simulink model "Comparacion"  (R2018a)
settings: Solver=VariableStepAuto  StartTime=0.0  StopTime=500  FixedStep=0.5  RelTol=1e-3
values from neighbouring files (symbols this model uses):
  A = [S.A zeros(n,p); -S.C eye(p)]    [poles_int.m]
  B = [S.B; zeros(p,m)]    [poles_int.m]
  q0 = eval(solucionParam.qs0)    [discretizacion.m]
  q1 = eval(solucionParam.qs1)    [discretizacion.m]
  q2 = eval(solucionParam.qs2)    [discretizacion.m]
  r1 = eval(solucionParam.rs1)    [discretizacion.m]
  ro = 0.0683    [LaplaceAzeta.m]    (also in discretizacion.m = 0.0683238685925)
  saturMax = 2    [discretizacion.m]
  saturMin = -.5    (= -0.5)    [discretizacion.m]
  so = 0.3356    [LaplaceAzeta.m]    (also in discretizacion.m = 0.335599308431)
  uo = 0.12    [LaplaceAzeta.m]    (also in discretizacion.m)
libraries: simulink x4
settings Model: Creator=posoriol1  LastModifiedBy=posoriol1

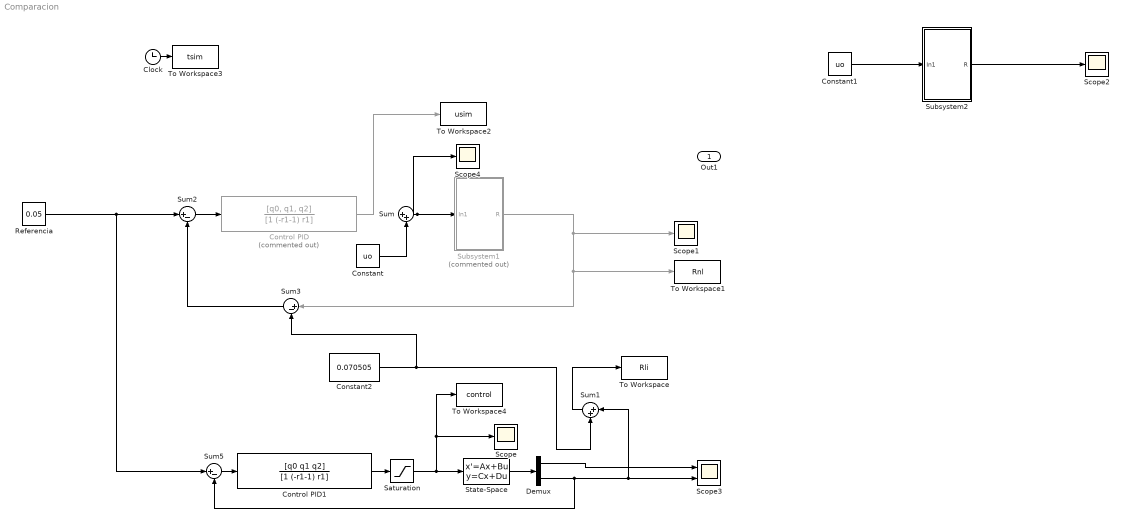
== system Comparacion ==
  Clock : Clock
  Constant : Constant  Value=uo  SampleTime=0.5
  Constant1 : Constant  Value=uo
  Constant2 : Constant  Value=0.070505
  Control PID : DiscreteTransferFcn  Commented=on  Numerator=[q0, q1, q2]  Denominator=[1 (-r1-1) r1]  SampleTime=0.5
  Control PID1 : DiscreteTransferFcn  Numerator=[q0 q1 q2]  Denominator=[1 (-r1-1) r1]  SampleTime=0.5
  Demux : Demux  Outputs=2
  Referencia : Constant  Value=0.05  SampleTime=0.5
  Saturation : Saturate  UpperLimit=saturMax  LowerLimit=saturMin
  Scope{,1..2,4} (4 alike) : Scope
  Scope3 : Scope  NumInputPorts=2
  State-Space : StateSpace  A=A  B=B  C=[1 0; 0 1]  D=[ 0;0]  InitialCondition=0
  Subsystem1 : Subsystem  Commented=on  mask{par=[0.14 0.1 0.3960 4^(-3) 0.2 0.09 0.0083], x0=[so, ro]}
      mask prompts: par "[bs br alphas q ms mr mc]"; x0 "Cond iniciales (s0,r0)"
      mask init:
      | bs=par(1);br=par(2);alphas=par(3);q=par(4);ms=par(5);mr=par(6);mc=par(7);
  Subsystem2 : Subsystem  mask{par=[0.14,0.1,0.3960,4^(-3),0.2,0.09,0.0083], x0=[so, ro]}
      mask prompts: par "[bs br alphas q ms mr mc]"; x0 "Cond iniciales (s0,r0)"
      mask init:
      | bs=par(1);br=par(2);alphas=par(3);q=par(4);ms=par(5);mr=par(6);mc=par(7);
  Sum : Sum  Inputs=|++
  Sum1 : Sum  Inputs=|++
  Sum2 : Sum  Inputs=|+-
  Sum3 : Sum  Inputs=|+-
  Sum5 : Sum  Inputs=|+-
  To Workspace : ToWorkspace  VariableName=Rli  SampleTime=-1
  To Workspace1 : ToWorkspace  VariableName=Rnl  SampleTime=-1
  To Workspace2 : ToWorkspace  VariableName=usim  SampleTime=-1
  To Workspace3 : ToWorkspace  VariableName=tsim  SampleTime=-1
  To Workspace4 : ToWorkspace  VariableName=control  SampleTime=-1
  Out1 : Outport
  wires:
  Referencia/1 -> Sum2/1, Sum5/1
  Constant2/1 -> Sum3/2, Sum1/2
  Sum5/1 -> Control PID1/1
  Sum1/1 -> To Workspace/1
  Constant/1 -> Sum/2
  Clock/1 -> To Workspace3/1
  Sum/1 -> Scope4/1, Subsystem1/1(In1)
  Control PID/1 -> To Workspace2/1
  Sum2/1 -> Control PID/1
  Constant1/1 -> Subsystem2/1(In1)
  Subsystem2/1(R) -> Scope2/1
  Subsystem1/1(R) -> Sum3/1, To Workspace1/1, Scope1/1
  Sum3/1 -> Sum2/2
  Control PID1/1 -> Saturation/1
  Saturation/1 -> Scope/1, To Workspace4/1, State-Space/1
  State-Space/1 -> Demux/1
  Demux/2 -> Sum5/2, Sum1/1, Scope3/2
  Demux/1 -> Scope3/1

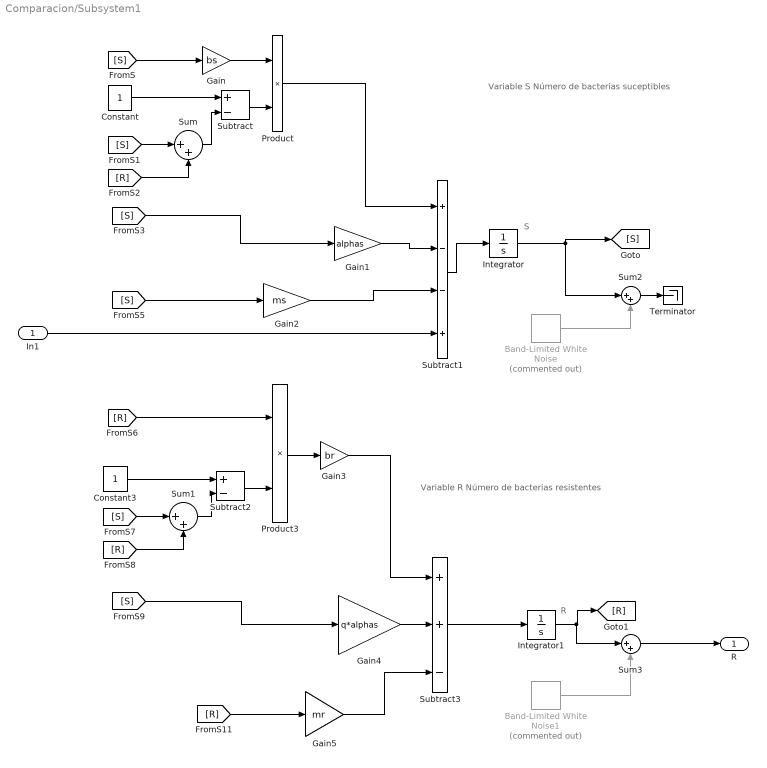
== system Comparacion/Subsystem1 ==
  note: R
  note: S
  note: Variable S
      | Número de bacterias suceptibles
  note: Variable R
      | Número de bacterias resistentes
  In1 : Inport
  Band-Limited White Noise : simulink/Sources/Band-Limited White Noise  Commented=on  Cov=[0.000001/100]  Ts=0.3  seed=[23341]
  Band-Limited White Noise1 : simulink/Sources/Band-Limited White Noise  Commented=on  Cov=[0.0000005/100]  Ts=0.3  seed=[11558]
  Constant : Constant
  Constant3 : Constant
  Gain : Gain  Gain=bs
  Gain1 : Gain  Gain=alphas
  Gain2 : Gain  Gain=ms
  Gain3 : Gain  Gain=br
  Gain4 : Gain  Gain=q*alphas
  Gain5 : Gain  Gain=mr
  Integrator : Integrator  InitialCondition=x0(1)
  Integrator1 : Integrator  InitialCondition=x0(2)
  Product : Product
  Product3 : Product
  Subtract : Sum  Inputs=+-
  Subtract1 : Sum  Inputs=+--+
  Subtract2 : Sum  Inputs=+-
  Subtract3 : Sum  Inputs=++-
  Sum{,1..3} (4 alike) : Sum  Inputs=|++
  Terminator : Terminator
  R : Outport
  wires:
  [S] -> Sum/1
  [R] -> Sum/2
  Constant/1 -> Subtract/1
  [S] -> Sum1/1
  Sum1/1 -> Subtract2/2
  Subtract1/1 -> Integrator/1
  Integrator/1 -> [S], Sum2/1
  [R] -> Sum1/2
  Constant3/1 -> Subtract2/1
  Product3/1 -> Gain3/1
  Product/1 -> Subtract1/1
  Integrator1/1 -> Sum3/1, [R]
  Subtract3/1 -> Integrator1/1
  Sum/1 -> Subtract/2
  [S] -> Gain/1
  Gain/1 -> Product/1
  Subtract/1 -> Product/2
  [S] -> Gain1/1
  Gain1/1 -> Subtract1/2
  [S] -> Gain2/1
  Gain2/1 -> Subtract1/3
  Gain3/1 -> Subtract3/1
  [R] -> Product3/1
  Subtract2/1 -> Product3/2
  Gain4/1 -> Subtract3/2
  [S] -> Gain4/1
  Gain5/1 -> Subtract3/3
  [R] -> Gain5/1
  In1/1 -> Subtract1/4
  Band-Limited White Noise/1 -> Sum2/2
  Band-Limited White Noise1/1 -> Sum3/2
  Sum3/1 -> R/1
  Sum2/1 -> Terminator/1

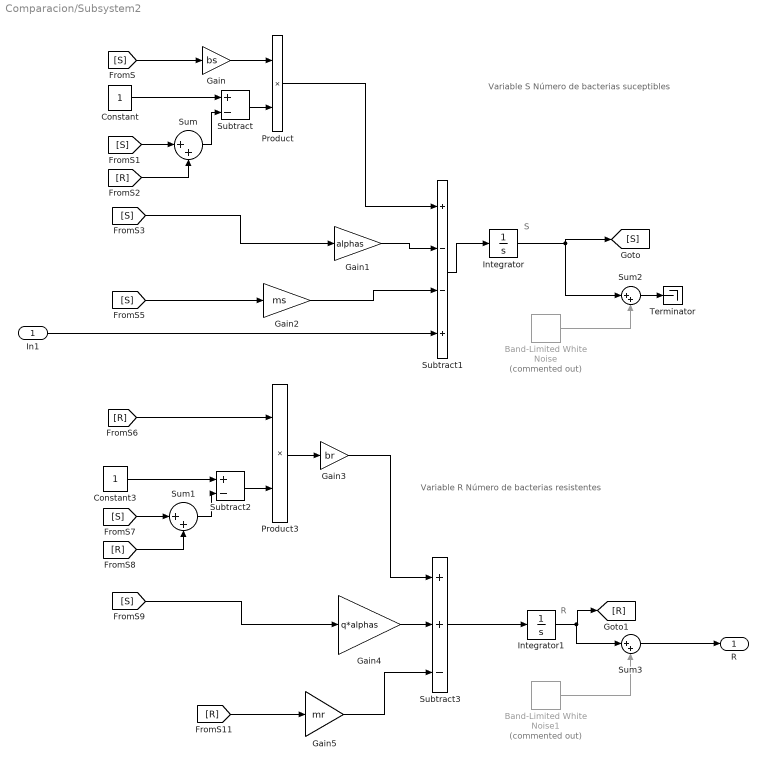
== system Comparacion/Subsystem2 ==
  note: R
  note: S
  note: Variable S
      | Número de bacterias suceptibles
  note: Variable R
      | Número de bacterias resistentes
  In1 : Inport
  Band-Limited White Noise : simulink/Sources/Band-Limited White Noise  Commented=on  Cov=[0.000001/100]  Ts=0.3  seed=[23341]
  Band-Limited White Noise1 : simulink/Sources/Band-Limited White Noise  Commented=on  Cov=[0.0000005/100]  Ts=0.3  seed=[11558]
  Constant : Constant
  Constant3 : Constant
  Gain : Gain  Gain=bs
  Gain1 : Gain  Gain=alphas
  Gain2 : Gain  Gain=ms
  Gain3 : Gain  Gain=br
  Gain4 : Gain  Gain=q*alphas
  Gain5 : Gain  Gain=mr
  Integrator : Integrator  InitialCondition=x0(1)
  Integrator1 : Integrator  InitialCondition=x0(2)
  Product : Product
  Product3 : Product
  Subtract : Sum  Inputs=+-
  Subtract1 : Sum  Inputs=+--+
  Subtract2 : Sum  Inputs=+-
  Subtract3 : Sum  Inputs=++-
  Sum{,1..3} (4 alike) : Sum  Inputs=|++
  Terminator : Terminator
  R : Outport
  wires:
  [S] -> Sum/1
  [R] -> Sum/2
  Constant/1 -> Subtract/1
  [S] -> Sum1/1
  Sum1/1 -> Subtract2/2
  Subtract1/1 -> Integrator/1
  Integrator/1 -> [S], Sum2/1
  [R] -> Sum1/2
  Constant3/1 -> Subtract2/1
  Product3/1 -> Gain3/1
  Product/1 -> Subtract1/1
  Integrator1/1 -> Sum3/1, [R]
  Subtract3/1 -> Integrator1/1
  Sum/1 -> Subtract/2
  [S] -> Gain/1
  Gain/1 -> Product/1
  Subtract/1 -> Product/2
  [S] -> Gain1/1
  Gain1/1 -> Subtract1/2
  [S] -> Gain2/1
  Gain2/1 -> Subtract1/3
  Gain3/1 -> Subtract3/1
  [R] -> Product3/1
  Subtract2/1 -> Product3/2
  Gain4/1 -> Subtract3/2
  [S] -> Gain4/1
  Gain5/1 -> Subtract3/3
  [R] -> Gain5/1
  In1/1 -> Subtract1/4
  Band-Limited White Noise/1 -> Sum2/2
  Band-Limited White Noise1/1 -> Sum3/2
  Sum3/1 -> R/1
  Sum2/1 -> Terminator/1
